simulink model "comp_dac_model"  (R2022a)
settings: Solver=VariableStepAuto  StartTime=0.0  StopTime=Tsim  RelTol=1e-3
values from neighbouring files (symbols this model uses):
  Fin = 15    [sim_comp_dac_model.m]
  fo = fsH/2    (= 48000000)    [sim_comp_dac_model.m]
  fsH = 96e6    (= 96000000)    [sim_comp_dac_model.m]
  h_comp_DAC = [-1/16 1-2^-3 -1/16]    [conf_comp_dac.m]
  switch_case = 2    [sim_comp_dac_model.m]
libraries: dspsrcs4 x2
settings Model: Creator=asper  LastModifiedBy=asper
settings ModelReferenceCC: EnableRefExpFcnMdlSchedulingChecks=off
settings RTWCC: Description=Generic Real-Time Target

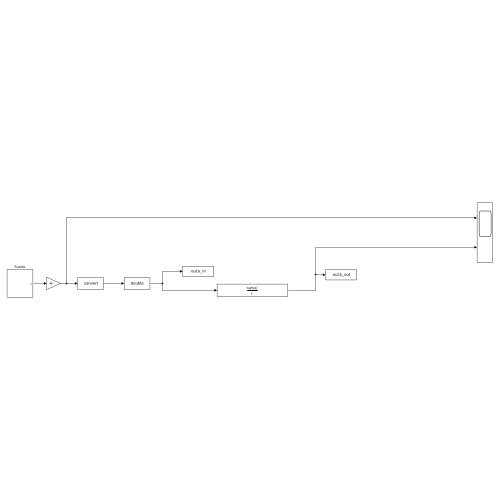
[thumbnail: Simulink's stored preview of the top-level diagram]
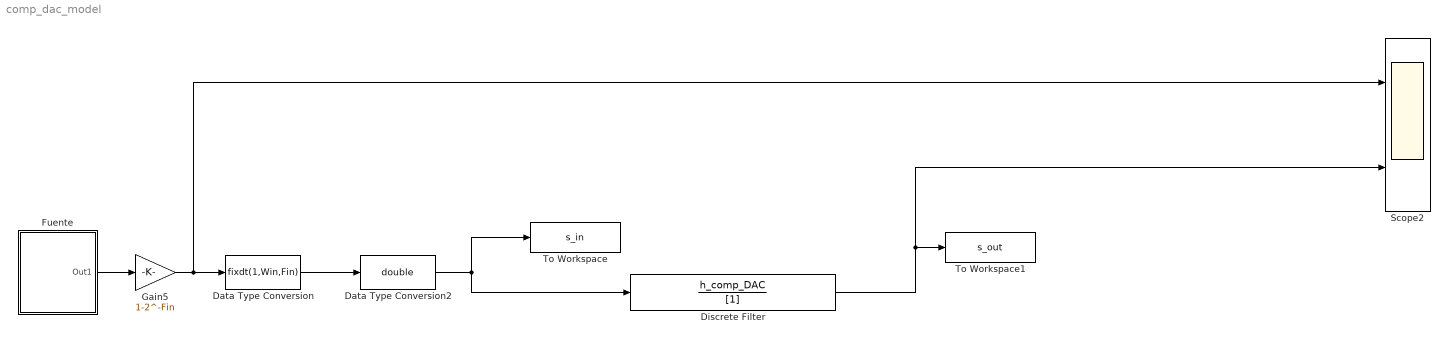
== system comp_dac_model ==
  Data Type Conversion : DataTypeConversion  OutDataTypeStr=fixdt(1,Win,Fin)  SaturateOnIntegerOverflow=off  RndMeth=Floor
  Data Type Conversion2 : DataTypeConversion  OutDataTypeStr=double  SaturateOnIntegerOverflow=off  RndMeth=Floor
  Discrete Filter : DiscreteFilter  Numerator=h_comp_DAC  Denominator=[1]
  Fuente : Subsystem
  Gain5 : Gain  Gain=1-2^-Fin
  Scope2 : Scope  NumInputPorts=2
  To Workspace : ToWorkspace  VariableName=s_in  SampleTime=-1
      settings: Save2DSignal=2-D array (concatenate along first dimension)
  To Workspace1 : ToWorkspace  VariableName=s_out  SampleTime=-1
      settings: Save2DSignal=2-D array (concatenate along first dimension)
  wires:
  Fuente/1(Out1) -> Gain5/1
  Gain5/1 -> Scope2/1, Data Type Conversion/1
  Data Type Conversion/1 -> Data Type Conversion2/1
  Discrete Filter/1 -> To Workspace1/1, Scope2/2
  Data Type Conversion2/1 -> To Workspace/1, Discrete Filter/1

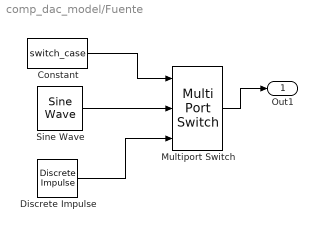
== system comp_dac_model/Fuente ==
  Constant : Constant  Value=switch_case
  Discrete Impulse : dspsrcs4/Discrete  Impulse  Delay=0  SampleTime=1/fsH  FrameSample=1  OutputFrames=off  dataType=double  isSigned=on  wordLen=16  udDataType=sfix(16)  fracBitsMode=Best precision  numFracBits=15  OutDataTypeStr=double  LastOutDataTypeStr=double
  Multiport Switch : MultiPortSwitch  Inputs=2  SaturateOnIntegerOverflow=off  InputSameDT=off
  Sine Wave : dspsrcs4/Sine Wave  Amplitude=1  Frequency=fo  Phase=0  SampleMode=Discrete  OutComplex=Real  CompMethod=Trigonometric fcn  TableSize=Speed  SampleTime=1/fsH  SamplesPerFrame=1  ResetState=Restart at time zero  OutputFrames=on  dataType=double  wordLen=16  udDataType=sfix(16)  fracBitsMode=User-defined  numFracBits=15  OutDataTypeStr=double  LastOutDataTypeStr=double
  Out1 : Outport  VectorParamsAs1DForOutWhenUnconnected=off
  wires:
  Multiport Switch/1 -> Out1/1
  Sine Wave/1 -> Multiport Switch/2
  Constant/1 -> Multiport Switch/1
  Discrete Impulse/1 -> Multiport Switch/3
